simulink model "souk_single_pipeline_4x2"  (R2021a)
settings: Solver=VariableStepAuto  StartTime=0.0  StopTime=10.0  RelTol=1e-3
undefined symbols (not defined in the file): datetime, posixtime
libraries: xbsIndex_r4 x9016, casper_library_misc x75, casper_library_delays x33, casper_library_reorder x22, xps_library x10
(part 16 of 104)

== system souk_single_pipeline_4x2/common/adc_ss/tt_lsb ==
  out_reg : Inport
  assert_reg : xbsIndex_r4/Assert  assert_type=on  type_source=Explicitly  gui_display_data_type=Fixed-point  arith_type=Unsigned  n_bits=32  bin_pt=0  preci_type=Single  exp_width=8  frac_width=24  assert_rate=off  rate_source=Explicitly  period=1  output_port=on  block_type=assert
  cast_gw : xbsIndex_r4/Convert  gui_display_data_type=Fixed-point  arith_type=Unsigned  n_bits=32  bin_pt=0  float_type=Single  exp_bits=8  fraction_bits=24  quantization=Truncate  overflow=Wrap  en=off  latency=1  pipeline=off  dbl_ovrd=off  block_type=convert
  io_delay : xbsIndex_r4/Delay  rst=off  infoeditControl=Selection of Reset will increase slice count due to use of real FFs and instead of SRLs  en=off  latency=0  reg_retiming=on  dbl_ovrd=off  block_type=delay
  reint1 : xbsIndex_r4/Reinterpret  force_arith_type=on  arith_type=Unsigned  force_bin_pt=on  bin_pt=0  block_type=reinterpret
  sim_out : Terminator
  sim_out_reg_gw : xbsIndex_r4/Gateway Out  inherit_from_input=off  hdl_port=off  rows=1  columns=1  UseAsDAC=off  DACChannel='1'  interface=None  automatic_assignment=on  address_offset=hex2dec('00')  intf_name=''  intf_description=''  timing_constraint=None  locs_specified=off  LOCs={}  io_standard={}  block_type=gatewayout
  sim_out_reg_sim_delay : xbsIndex_r4/Delay  rst=off  infoeditControl=Selection of Reset will increase slice count due to use of real FFs and instead of SRLs  en=off  latency=1  reg_retiming=on  dbl_ovrd=off  block_type=delay
  souk_single_pipeline_4x2_common_adc_ss_tt_lsb_user_data_in : xbsIndex_r4/Gateway Out  inherit_from_input=off  hdl_port=on  rows=1  columns=1  UseAsDAC=off  DACChannel='1'  interface=None  automatic_assignment=on  address_offset=hex2dec('00')  intf_name=''  intf_description=''  timing_constraint=None  locs_specified=off  LOCs={}  io_standard={}  block_type=gatewayout
  sim_out_reg : Outport  VectorParamsAs1DForOutWhenUnconnected=off
  wires:
  sim_out_reg_sim_delay/1 -> sim_out_reg_gw/1
  sim_out_reg_gw/1 -> sim_out_reg/1
  io_delay/1 -> cast_gw/1
  cast_gw/1 -> souk_single_pipeline_4x2_common_adc_ss_tt_lsb_user_data_in/1
  souk_single_pipeline_4x2_common_adc_ss_tt_lsb_user_data_in/1 -> sim_out/1
  out_reg/1 -> sim_out_reg_sim_delay/1, assert_reg/1
  assert_reg/1 -> reint1/1
  reint1/1 -> io_delay/1

== system souk_single_pipeline_4x2/common/adc_ss/tt_msb ==
  out_reg : Inport
  assert_reg : xbsIndex_r4/Assert  assert_type=on  type_source=Explicitly  gui_display_data_type=Fixed-point  arith_type=Unsigned  n_bits=32  bin_pt=0  preci_type=Single  exp_width=8  frac_width=24  assert_rate=off  rate_source=Explicitly  period=1  output_port=on  block_type=assert
  cast_gw : xbsIndex_r4/Convert  gui_display_data_type=Fixed-point  arith_type=Unsigned  n_bits=32  bin_pt=0  float_type=Single  exp_bits=8  fraction_bits=24  quantization=Truncate  overflow=Wrap  en=off  latency=1  pipeline=off  dbl_ovrd=off  block_type=convert
  io_delay : xbsIndex_r4/Delay  rst=off  infoeditControl=Selection of Reset will increase slice count due to use of real FFs and instead of SRLs  en=off  latency=0  reg_retiming=on  dbl_ovrd=off  block_type=delay
  reint1 : xbsIndex_r4/Reinterpret  force_arith_type=on  arith_type=Unsigned  force_bin_pt=on  bin_pt=0  block_type=reinterpret
  sim_out : Terminator
  sim_out_reg_gw : xbsIndex_r4/Gateway Out  inherit_from_input=off  hdl_port=off  rows=1  columns=1  UseAsDAC=off  DACChannel='1'  interface=None  automatic_assignment=on  address_offset=hex2dec('00')  intf_name=''  intf_description=''  timing_constraint=None  locs_specified=off  LOCs={}  io_standard={}  block_type=gatewayout
  sim_out_reg_sim_delay : xbsIndex_r4/Delay  rst=off  infoeditControl=Selection of Reset will increase slice count due to use of real FFs and instead of SRLs  en=off  latency=1  reg_retiming=on  dbl_ovrd=off  block_type=delay
  souk_single_pipeline_4x2_common_adc_ss_tt_msb_user_data_in : xbsIndex_r4/Gateway Out  inherit_from_input=off  hdl_port=on  rows=1  columns=1  UseAsDAC=off  DACChannel='1'  interface=None  automatic_assignment=on  address_offset=hex2dec('00')  intf_name=''  intf_description=''  timing_constraint=None  locs_specified=off  LOCs={}  io_standard={}  block_type=gatewayout
  sim_out_reg : Outport  VectorParamsAs1DForOutWhenUnconnected=off
  wires:
  sim_out_reg_sim_delay/1 -> sim_out_reg_gw/1
  sim_out_reg_gw/1 -> sim_out_reg/1
  io_delay/1 -> cast_gw/1
  cast_gw/1 -> souk_single_pipeline_4x2_common_adc_ss_tt_msb_user_data_in/1
  souk_single_pipeline_4x2_common_adc_ss_tt_msb_user_data_in/1 -> sim_out/1
  out_reg/1 -> sim_out_reg_sim_delay/1, assert_reg/1
  assert_reg/1 -> reint1/1
  reint1/1 -> io_delay/1

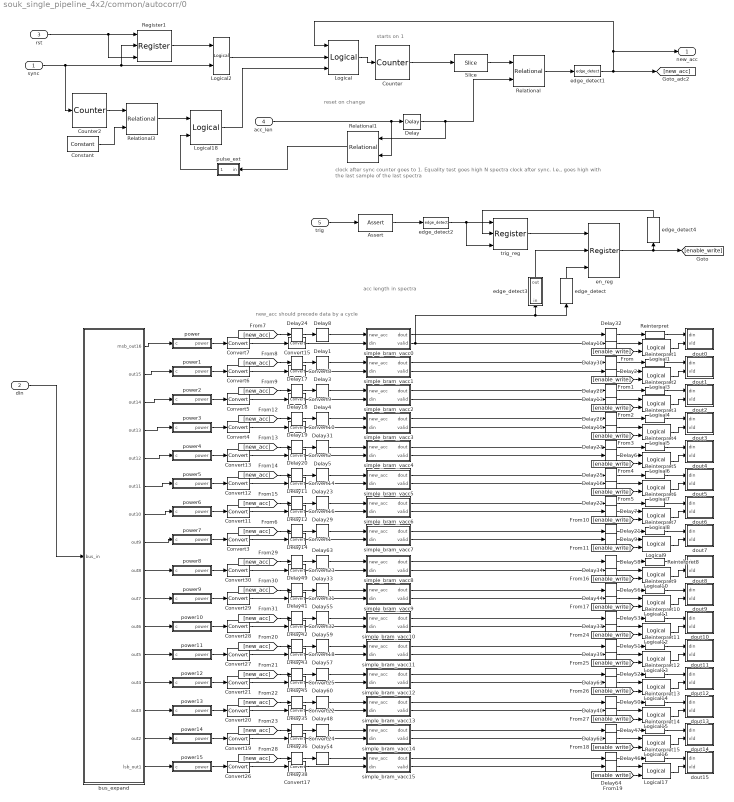
== system souk_single_pipeline_4x2/common/autocorr/0 ==
  note: reset on change
  note: starts on 1
  note: clock after sync counter goes to 1.
      |
      | Equality test goes high N spectra clock after sync. I.e., goes high with the last sample of the last spectra
  note: acc length in spectra
  note: new_acc should precede data by a cycle
  sync : Inport
  din : Inport  Port=2
  rst : Inport  Port=3
  acc_len : Inport  Port=4
  trig : Inport  Port=5
  Assert : xbsIndex_r4/Assert  assert_type=off  type_source=Explicitly  gui_display_data_type=Fixed-point  arith_type="Signed  (2's comp)"  n_bits=16  bin_pt=14  preci_type=Single  exp_width=8  frac_width=24  assert_rate=on  rate_source=Explicitly  period=1  output_port=on  block_type=assert
  Constant : xbsIndex_r4/Constant  const=2^(nchan_bits + npol_bits) - 1  gui_display_data_type=Fixed-point  arith_type=Unsigned  n_bits=nchan_bits + npol_bits  bin_pt=0  preci_type=Single  exp_width=8  frac_width=24  explicit_period=on  period=1  equ=P=C  opselect=C  inp2=PCIN>>17  opr=+  inp1=P  carry=CIN  dbl_ovrd=off  block_type=constant
  Convert{1..2,8..10,14..18,22..25,31..32} (16 alike) : xbsIndex_r4/Convert  gui_display_data_type=Floating-point  arith_type=Floating-point  n_bits=31  bin_pt=28  float_type=Single  exp_bits=8  fraction_bits=24  quantization="Round  (unbiased: Even Values)"  overflow=Wrap  en=off  latency=3  pipeline=on  dbl_ovrd=off  block_type=convert
  Convert{3..7,11..13,19..21,26..30} (16 alike) : xbsIndex_r4/Convert  gui_display_data_type=Fixed-point  arith_type="Signed  (2's comp)"  n_bits=37  bin_pt=34  float_type=Single  exp_bits=8  fraction_bits=24  quantization=Truncate  overflow=Wrap  en=off  latency=0  pipeline=off  dbl_ovrd=off  block_type=convert
  Counter : xbsIndex_r4/Counter  cnt_type=Free Running  cnt_to=Inf  operation=Up  start_count=1  cnt_by_val=1  arith_type=Unsigned  n_bits=30  bin_pt=0  load_pin=off  rst=on  en=off  explicit_period=on  period=1  use_behavioral_HDL=off  implementation=Fabric  dbl_ovrd=off  block_type=counter
  Counter2 : xbsIndex_r4/Counter  cnt_type=Free Running  cnt_to=Inf  operation=Up  start_count=0  cnt_by_val=1  arith_type=Unsigned  n_bits=nchan_bits + npol_bits  bin_pt=0  load_pin=off  rst=on  en=off  explicit_period=on  period=1  use_behavioral_HDL=off  implementation=Fabric  dbl_ovrd=off  block_type=counter
  Delay{,2,6..7,9..10,13,15..16,34,37,39..40,44,61..62,64} (17 alike) : xbsIndex_r4/Delay  rst=off  infoeditControl=Selection of Reset will increase slice count due to use of real FFs and instead of SRLs  en=off  latency=1  reg_retiming=off  dbl_ovrd=off  block_type=delay
  Delay{1,3..5,8,23,29,31,33,48,54..55,57,59..60,63} (16 alike) : xbsIndex_r4/Delay  rst=off  infoeditControl=Selection of Reset will increase slice count due to use of real FFs and instead of SRLs  en=off  latency=4  reg_retiming=on  dbl_ovrd=off  block_type=delay
  Delay{11..12,14,17..20,24,35..36,38,41..43,45,49} (16 alike) : xbsIndex_r4/Delay  rst=off  infoeditControl=Selection of Reset will increase slice count due to use of real FFs and instead of SRLs  en=off  latency=3  reg_retiming=on  dbl_ovrd=off  block_type=delay
  Delay{21..22,25..28,30,32,46..47,50..53,56,58} (16 alike) : xbsIndex_r4/Delay  rst=off  infoeditControl=Selection of Reset will increase slice count due to use of real FFs and instead of SRLs  en=off  latency=1  reg_retiming=on  dbl_ovrd=off  block_type=delay
  Logical : xbsIndex_r4/Logical  logical_function=OR  inputs=3  en=off  latency=0  precision=Full  arith_type=Unsigned  n_bits=16  bin_pt=0  align_bp=on  dbl_ovrd=off  block_type=logical
  Logical{1..18} (18 alike) : xbsIndex_r4/Logical  logical_function=AND  inputs=2  en=off  latency=0  precision=Full  arith_type=Unsigned  n_bits=16  bin_pt=0  align_bp=on  dbl_ovrd=off  block_type=logical
  Register1 : xbsIndex_r4/Register  init=0  rst=on  en=on  dbl_ovrd=off  block_type=register
  Reinterpret{,1..15} (16 alike) : xbsIndex_r4/Reinterpret  force_arith_type=on  arith_type=Unsigned  force_bin_pt=on  bin_pt=0  block_type=reinterpret
  Relational : xbsIndex_r4/Relational  mode=a=b  op_type=Bool  en=off  latency=0  dbl_ovrd=off  block_type=relational
  Relational1 : xbsIndex_r4/Relational  mode=a!=b  op_type=Bool  en=off  latency=1  dbl_ovrd=off  block_type=relational
  Relational3 : xbsIndex_r4/Relational  mode=a=b  op_type=Bool  en=off  latency=1  dbl_ovrd=off  block_type=relational
  Slice : xbsIndex_r4/Slice  nbits=30-nchan_bits-npol_bits  boolean_output=off  mode=Lower Bit Location + Width  bit1=0  base1=MSB of Input  bit0=nchan_bits + npol_bits  base0=LSB of Input  dbl_ovrd=off  block_type=slice
  bus_expand : Subsystem  AncestorBlock=casper_library_flow_control/bus_expand  mask(bus_expand){mode=divisions of equal size, outputNum=16, outputWidth=36, outputBinaryPt=0, outputArithmeticType=0, show_format=off, outputToWorkspace=off, variablePrefix=out, outputToModelAsWell=on}
      mask prompts: outputNum "Number of outputs:"; outputWidth "Output width:"; outputBinaryPt "Output binary point position:"; outputArithmeticType "Output arithmetic type (ufix=0, fix=1, bool=2):"; show_format "Print format string?"; outputToWorkspace "Output to workspace?"; variablePrefix "Variable name prefix:"; outputToModelAsWell "Output to model as well?"
      mask help:
      | Expands a 'bus' made using a bus_create or Xilinx
      | concat block.
      | The input will be divided into the specified number
      | of outputs with the specified arithmetic types.
      | Divisions are made from most significant bit.
      mask init: same as souk_single_pipeline_4x2/bus_expand
      settings: AttributesFormatString=16 outputs
      mask TypeOptions mode: divisions of equal size | divisions of arbitrary size
      mask Callback mode: %bus_expand_callback();
      mask Callback outputWidth: %bus_expand_callback();
      mask Callback outputToWorkspace: %bus_expand_callback();
  dout0 : Subsystem
  dout1 : Subsystem
  dout10 : Subsystem
  dout11 : Subsystem
  dout12 : Subsystem
  dout13 : Subsystem
  dout14 : Subsystem
  dout15 : Subsystem
  dout2 : Subsystem
  dout3 : Subsystem
  dout4 : Subsystem
  dout5 : Subsystem
  dout6 : Subsystem
  dout7 : Subsystem
  dout8 : Subsystem
  dout9 : Subsystem
  edge_detect{,1..2,4} (4 alike) : casper_library_misc/edge_detect  edge=Rising  polarity=Active High  x_in=[0 0.08 0.08 0.16 0.16 0.24 0.24 0.32 0.32 0.4]  y_in="[-1 -1  1  1  1  1  1  1  1  1]"  x_out=[0.6 0.68 0.68 0.76 0.76 0.84 0.84 0.92 0.92 1]  y_out="[-1 -1  1  1 -1 -1 -1 -1 -1 -1]"
  edge_detect3 : Subsystem  AncestorBlock=casper_library_misc/edge_detect  mask(edge_detect){edge=Falling, polarity=Active High, x_in=[0 0.08 0.08 0.16 0.16 0.24 0.24 0.32 0.32 0.4], y_in=[-1 -1  1  1  1  1  1  1  1  1], x_out=[0.6 0.68 0.68 0.76 0.76 0.84 0.84 0.92 0.92 1], y_out=[-1 -1  1  1 -1 -1 -1 -1 -1 -1]}
      mask prompts: edge "Edge Type"; polarity "Output Polarity"; x_in "Input X Positions"; y_in "Input Y Positions"; x_out "Output X Positions"; y_out "Output Y Positions"
      mask help: Output is active for one-cycle after each edge of the specified type (i.e. rising, falling or both).
      mask init: same as souk_single_pipeline_4x2/pulse_ext/posedge
      settings: AttributesFormatString=|
      | falling edges
      | active high
      mask Help: Output is active for one-cycle after each edge of the specified type (i.e. rising, falling, or both).  Latency is zero.
      mask TypeOptions edge: Rising | Falling | Both
      mask TypeOptions polarity: Active High | Active Low
      mask Display:
      | plot(x_in_num,0.5+y_in_num*0.2);
      | plot(x_out_num,0.5+y_out_num*0.2);
  en_reg : xbsIndex_r4/Register  init=0  rst=on  en=on  dbl_ovrd=off  block_type=register
  power : Subsystem  mask(power){BitWidth=18, add_latency=1, mult_latency=3}
      mask prompts: BitWidth "Bit Width"; add_latency "Add Latency"; mult_latency "Mult Latency"
      mask help: Squares real and imaginary components of complex input and adds them.
      mask Help: eval('xlWeb(''http://casper.berkeley.edu/wiki/Power'')')
      mask Display:
      | port_label('input', 1, 'c');
      | port_label('output', 1, 'power');
      | disp(['Z^-', num2str(mult_latency+add_latency)]);
  power1 : Subsystem  mask(power){BitWidth=18, add_latency=1, mult_latency=3}
      mask prompts: BitWidth "Bit Width"; add_latency "Add Latency"; mult_latency "Mult Latency"
      mask help: Squares real and imaginary components of complex input and adds them.
      mask Help: eval('xlWeb(''http://casper.berkeley.edu/wiki/Power'')')
      mask Display:
      | port_label('input', 1, 'c');
      | port_label('output', 1, 'power');
      | disp(['Z^-', num2str(mult_latency+add_latency)]);
  power10 : Subsystem  mask(power){BitWidth=18, add_latency=1, mult_latency=3}
      mask prompts: BitWidth "Bit Width"; add_latency "Add Latency"; mult_latency "Mult Latency"
      mask help: Squares real and imaginary components of complex input and adds them.
      mask Help: eval('xlWeb(''http://casper.berkeley.edu/wiki/Power'')')
      mask Display:
      | port_label('input', 1, 'c');
      | port_label('output', 1, 'power');
      | disp(['Z^-', num2str(mult_latency+add_latency)]);
  power11 : Subsystem  mask(power){BitWidth=18, add_latency=1, mult_latency=3}
      mask prompts: BitWidth "Bit Width"; add_latency "Add Latency"; mult_latency "Mult Latency"
      mask help: Squares real and imaginary components of complex input and adds them.
      mask Help: eval('xlWeb(''http://casper.berkeley.edu/wiki/Power'')')
      mask Display:
      | port_label('input', 1, 'c');
      | port_label('output', 1, 'power');
      | disp(['Z^-', num2str(mult_latency+add_latency)]);
  power12 : Subsystem  mask(power){BitWidth=18, add_latency=1, mult_latency=3}
      mask prompts: BitWidth "Bit Width"; add_latency "Add Latency"; mult_latency "Mult Latency"
      mask help: Squares real and imaginary components of complex input and adds them.
      mask Help: eval('xlWeb(''http://casper.berkeley.edu/wiki/Power'')')
      mask Display:
      | port_label('input', 1, 'c');
      | port_label('output', 1, 'power');
      | disp(['Z^-', num2str(mult_latency+add_latency)]);
  power13 : Subsystem  mask(power){BitWidth=18, add_latency=1, mult_latency=3}
      mask prompts: BitWidth "Bit Width"; add_latency "Add Latency"; mult_latency "Mult Latency"
      mask help: Squares real and imaginary components of complex input and adds them.
      mask Help: eval('xlWeb(''http://casper.berkeley.edu/wiki/Power'')')
      mask Display:
      | port_label('input', 1, 'c');
      | port_label('output', 1, 'power');
      | disp(['Z^-', num2str(mult_latency+add_latency)]);
  power14 : Subsystem  mask(power){BitWidth=18, add_latency=1, mult_latency=3}
      mask prompts: BitWidth "Bit Width"; add_latency "Add Latency"; mult_latency "Mult Latency"
      mask help: Squares real and imaginary components of complex input and adds them.
      mask Help: eval('xlWeb(''http://casper.berkeley.edu/wiki/Power'')')
      mask Display:
      | port_label('input', 1, 'c');
      | port_label('output', 1, 'power');
      | disp(['Z^-', num2str(mult_latency+add_latency)]);
  power15 : Subsystem  mask(power){BitWidth=18, add_latency=1, mult_latency=3}
      mask prompts: BitWidth "Bit Width"; add_latency "Add Latency"; mult_latency "Mult Latency"
      mask help: Squares real and imaginary components of complex input and adds them.
      mask Help: eval('xlWeb(''http://casper.berkeley.edu/wiki/Power'')')
      mask Display:
      | port_label('input', 1, 'c');
      | port_label('output', 1, 'power');
      | disp(['Z^-', num2str(mult_latency+add_latency)]);
  power2 : Subsystem  mask(power){BitWidth=18, add_latency=1, mult_latency=3}
      mask prompts: BitWidth "Bit Width"; add_latency "Add Latency"; mult_latency "Mult Latency"
      mask help: Squares real and imaginary components of complex input and adds them.
      mask Help: eval('xlWeb(''http://casper.berkeley.edu/wiki/Power'')')
      mask Display:
      | port_label('input', 1, 'c');
      | port_label('output', 1, 'power');
      | disp(['Z^-', num2str(mult_latency+add_latency)]);
  power3 : Subsystem  mask(power){BitWidth=18, add_latency=1, mult_latency=3}
      mask prompts: BitWidth "Bit Width"; add_latency "Add Latency"; mult_latency "Mult Latency"
      mask help: Squares real and imaginary components of complex input and adds them.
      mask Help: eval('xlWeb(''http://casper.berkeley.edu/wiki/Power'')')
      mask Display:
      | port_label('input', 1, 'c');
      | port_label('output', 1, 'power');
      | disp(['Z^-', num2str(mult_latency+add_latency)]);
  power4 : Subsystem  mask(power){BitWidth=18, add_latency=1, mult_latency=3}
      mask prompts: BitWidth "Bit Width"; add_latency "Add Latency"; mult_latency "Mult Latency"
      mask help: Squares real and imaginary components of complex input and adds them.
      mask Help: eval('xlWeb(''http://casper.berkeley.edu/wiki/Power'')')
      mask Display:
      | port_label('input', 1, 'c');
      | port_label('output', 1, 'power');
      | disp(['Z^-', num2str(mult_latency+add_latency)]);
  power5 : Subsystem  mask(power){BitWidth=18, add_latency=1, mult_latency=3}
      mask prompts: BitWidth "Bit Width"; add_latency "Add Latency"; mult_latency "Mult Latency"
      mask help: Squares real and imaginary components of complex input and adds them.
      mask Help: eval('xlWeb(''http://casper.berkeley.edu/wiki/Power'')')
      mask Display:
      | port_label('input', 1, 'c');
      | port_label('output', 1, 'power');
      | disp(['Z^-', num2str(mult_latency+add_latency)]);
  power6 : Subsystem  mask(power){BitWidth=18, add_latency=1, mult_latency=3}
      mask prompts: BitWidth "Bit Width"; add_latency "Add Latency"; mult_latency "Mult Latency"
      mask help: Squares real and imaginary components of complex input and adds them.
      mask Help: eval('xlWeb(''http://casper.berkeley.edu/wiki/Power'')')
      mask Display:
      | port_label('input', 1, 'c');
      | port_label('output', 1, 'power');
      | disp(['Z^-', num2str(mult_latency+add_latency)]);
  power7 : Subsystem  mask(power){BitWidth=18, add_latency=1, mult_latency=3}
      mask prompts: BitWidth "Bit Width"; add_latency "Add Latency"; mult_latency "Mult Latency"
      mask help: Squares real and imaginary components of complex input and adds them.
      mask Help: eval('xlWeb(''http://casper.berkeley.edu/wiki/Power'')')
      mask Display:
      | port_label('input', 1, 'c');
      | port_label('output', 1, 'power');
      | disp(['Z^-', num2str(mult_latency+add_latency)]);
  power8 : Subsystem  mask(power){BitWidth=18, add_latency=1, mult_latency=3}
      mask prompts: BitWidth "Bit Width"; add_latency "Add Latency"; mult_latency "Mult Latency"
      mask help: Squares real and imaginary components of complex input and adds them.
      mask Help: eval('xlWeb(''http://casper.berkeley.edu/wiki/Power'')')
      mask Display:
      | port_label('input', 1, 'c');
      | port_label('output', 1, 'power');
      | disp(['Z^-', num2str(mult_latency+add_latency)]);
  power9 : Subsystem  mask(power){BitWidth=18, add_latency=1, mult_latency=3}
      mask prompts: BitWidth "Bit Width"; add_latency "Add Latency"; mult_latency "Mult Latency"
      mask help: Squares real and imaginary components of complex input and adds them.
      mask Help: eval('xlWeb(''http://casper.berkeley.edu/wiki/Power'')')
      mask Display:
      | port_label('input', 1, 'c');
      | port_label('output', 1, 'power');
      | disp(['Z^-', num2str(mult_latency+add_latency)]);
  pulse_ext : Subsystem  AncestorBlock=casper_library_misc/pulse_ext  mask(pulse_ext){pulse_len=2^(nchan_bits + npol_bits)}
      mask prompts: pulse_len "Length of Pulse"
      mask help:
      | Extends a boolean signal to be high for the specified number of clocks after
      | the last high input.
      mask init:
      | bits = ceil(log2(pulse_len+1));
      mask Help: eval('xlWeb(''http://casper.berkeley.edu/wiki/Pulse_ext'')')
  simple_bram_vacc0 : Subsystem  AncestorBlock=casper_library_accumulators/simple_bram_vacc  mask(simple_bram_vacc){vec_len=2^(nchan_bits + npol_bits), arith_type=Signed, n_bits=30 + 17, bin_pt=28}
      mask prompts: vec_len "Vector length:"; arith_type "Output type:"; n_bits "Bit width (output):"; bin_pt "Binary point (output):"
      mask help: This simple vector accumulator is based on a shift register. It outputs its previous accumulated vector after a new_acc pulse is received.
      mask init:
      | simple_bram_vacc_init(gcb, ...
      |     'vec_len', vec_len, ...
      |     'arith_type', arith_type, ...
      |     'n_bits', n_bits, ...
      |     'bin_pt', bin_pt);
      mask TypeOptions arith_type: Signed | Unsigned
  simple_bram_vacc1 : Subsystem  AncestorBlock=casper_library_accumulators/simple_bram_vacc  mask(simple_bram_vacc){vec_len=2^(nchan_bits + npol_bits), arith_type=Signed, n_bits=30 + 17, bin_pt=28}
      mask prompts: vec_len "Vector length:"; arith_type "Output type:"; n_bits "Bit width (output):"; bin_pt "Binary point (output):"
      mask help: This simple vector accumulator is based on a shift register. It outputs its previous accumulated vector after a new_acc pulse is received.
      mask init:
      | simple_bram_vacc_init(gcb, ...
      |     'vec_len', vec_len, ...
      |     'arith_type', arith_type, ...
      |     'n_bits', n_bits, ...
      |     'bin_pt', bin_pt);
      mask TypeOptions arith_type: Signed | Unsigned
  simple_bram_vacc10 : Subsystem  AncestorBlock=casper_library_accumulators/simple_bram_vacc  mask(simple_bram_vacc){vec_len=2^(nchan_bits + npol_bits), arith_type=Signed, n_bits=30 + 17, bin_pt=28}
      mask prompts: vec_len "Vector length:"; arith_type "Output type:"; n_bits "Bit width (output):"; bin_pt "Binary point (output):"
      mask help: This simple vector accumulator is based on a shift register. It outputs its previous accumulated vector after a new_acc pulse is received.
      mask init:
      | simple_bram_vacc_init(gcb, ...
      |     'vec_len', vec_len, ...
      |     'arith_type', arith_type, ...
      |     'n_bits', n_bits, ...
      |     'bin_pt', bin_pt);
      mask TypeOptions arith_type: Signed | Unsigned
  simple_bram_vacc11 : Subsystem  AncestorBlock=casper_library_accumulators/simple_bram_vacc  mask(simple_bram_vacc){vec_len=2^(nchan_bits + npol_bits), arith_type=Signed, n_bits=30 + 17, bin_pt=28}
      mask prompts: vec_len "Vector length:"; arith_type "Output type:"; n_bits "Bit width (output):"; bin_pt "Binary point (output):"
      mask help: This simple vector accumulator is based on a shift register. It outputs its previous accumulated vector after a new_acc pulse is received.
      mask init:
      | simple_bram_vacc_init(gcb, ...
      |     'vec_len', vec_len, ...
      |     'arith_type', arith_type, ...
      |     'n_bits', n_bits, ...
      |     'bin_pt', bin_pt);
      mask TypeOptions arith_type: Signed | Unsigned
  simple_bram_vacc12 : Subsystem  AncestorBlock=casper_library_accumulators/simple_bram_vacc  mask(simple_bram_vacc){vec_len=2^(nchan_bits + npol_bits), arith_type=Signed, n_bits=30 + 17, bin_pt=28}
      mask prompts: vec_len "Vector length:"; arith_type "Output type:"; n_bits "Bit width (output):"; bin_pt "Binary point (output):"
      mask help: This simple vector accumulator is based on a shift register. It outputs its previous accumulated vector after a new_acc pulse is received.
      mask init:
      | simple_bram_vacc_init(gcb, ...
      |     'vec_len', vec_len, ...
      |     'arith_type', arith_type, ...
      |     'n_bits', n_bits, ...
      |     'bin_pt', bin_pt);
      mask TypeOptions arith_type: Signed | Unsigned
  simple_bram_vacc13 : Subsystem  AncestorBlock=casper_library_accumulators/simple_bram_vacc  mask(simple_bram_vacc){vec_len=2^(nchan_bits + npol_bits), arith_type=Signed, n_bits=30 + 17, bin_pt=28}
      mask prompts: vec_len "Vector length:"; arith_type "Output type:"; n_bits "Bit width (output):"; bin_pt "Binary point (output):"
      mask help: This simple vector accumulator is based on a shift register. It outputs its previous accumulated vector after a new_acc pulse is received.
      mask init:
      | simple_bram_vacc_init(gcb, ...
      |     'vec_len', vec_len, ...
      |     'arith_type', arith_type, ...
      |     'n_bits', n_bits, ...
      |     'bin_pt', bin_pt);
      mask TypeOptions arith_type: Signed | Unsigned
  simple_bram_vacc14 : Subsystem  AncestorBlock=casper_library_accumulators/simple_bram_vacc  mask(simple_bram_vacc){vec_len=2^(nchan_bits + npol_bits), arith_type=Signed, n_bits=30 + 17, bin_pt=28}
      mask prompts: vec_len "Vector length:"; arith_type "Output type:"; n_bits "Bit width (output):"; bin_pt "Binary point (output):"
      mask help: This simple vector accumulator is based on a shift register. It outputs its previous accumulated vector after a new_acc pulse is received.
      mask init:
      | simple_bram_vacc_init(gcb, ...
      |     'vec_len', vec_len, ...
      |     'arith_type', arith_type, ...
      |     'n_bits', n_bits, ...
      |     'bin_pt', bin_pt);
      mask TypeOptions arith_type: Signed | Unsigned
  simple_bram_vacc15 : Subsystem  AncestorBlock=casper_library_accumulators/simple_bram_vacc  mask(simple_bram_vacc){vec_len=2^(nchan_bits + npol_bits), arith_type=Signed, n_bits=30 + 17, bin_pt=28}
      mask prompts: vec_len "Vector length:"; arith_type "Output type:"; n_bits "Bit width (output):"; bin_pt "Binary point (output):"
      mask help: This simple vector accumulator is based on a shift register. It outputs its previous accumulated vector after a new_acc pulse is received.
      mask init:
      | simple_bram_vacc_init(gcb, ...
      |     'vec_len', vec_len, ...
      |     'arith_type', arith_type, ...
      |     'n_bits', n_bits, ...
      |     'bin_pt', bin_pt);
      mask TypeOptions arith_type: Signed | Unsigned
  simple_bram_vacc2 : Subsystem  AncestorBlock=casper_library_accumulators/simple_bram_vacc  mask(simple_bram_vacc){vec_len=2^(nchan_bits + npol_bits), arith_type=Signed, n_bits=30 + 17, bin_pt=28}
      mask prompts: vec_len "Vector length:"; arith_type "Output type:"; n_bits "Bit width (output):"; bin_pt "Binary point (output):"
      mask help: This simple vector accumulator is based on a shift register. It outputs its previous accumulated vector after a new_acc pulse is received.
      mask init:
      | simple_bram_vacc_init(gcb, ...
      |     'vec_len', vec_len, ...
      |     'arith_type', arith_type, ...
      |     'n_bits', n_bits, ...
      |     'bin_pt', bin_pt);
      mask TypeOptions arith_type: Signed | Unsigned
  simple_bram_vacc3 : Subsystem  AncestorBlock=casper_library_accumulators/simple_bram_vacc  mask(simple_bram_vacc){vec_len=2^(nchan_bits + npol_bits), arith_type=Signed, n_bits=30 + 17, bin_pt=28}
      mask prompts: vec_len "Vector length:"; arith_type "Output type:"; n_bits "Bit width (output):"; bin_pt "Binary point (output):"
      mask help: This simple vector accumulator is based on a shift register. It outputs its previous accumulated vector after a new_acc pulse is received.
      mask init:
      | simple_bram_vacc_init(gcb, ...
      |     'vec_len', vec_len, ...
      |     'arith_type', arith_type, ...
      |     'n_bits', n_bits, ...
      |     'bin_pt', bin_pt);
      mask TypeOptions arith_type: Signed | Unsigned
  simple_bram_vacc4 : Subsystem  AncestorBlock=casper_library_accumulators/simple_bram_vacc  mask(simple_bram_vacc){vec_len=2^(nchan_bits + npol_bits), arith_type=Signed, n_bits=30 + 17, bin_pt=28}
      mask prompts: vec_len "Vector length:"; arith_type "Output type:"; n_bits "Bit width (output):"; bin_pt "Binary point (output):"
      mask help: This simple vector accumulator is based on a shift register. It outputs its previous accumulated vector after a new_acc pulse is received.
      mask init:
      | simple_bram_vacc_init(gcb, ...
      |     'vec_len', vec_len, ...
      |     'arith_type', arith_type, ...
      |     'n_bits', n_bits, ...
      |     'bin_pt', bin_pt);
      mask TypeOptions arith_type: Signed | Unsigned
  simple_bram_vacc5 : Subsystem  AncestorBlock=casper_library_accumulators/simple_bram_vacc  mask(simple_bram_vacc){vec_len=2^(nchan_bits + npol_bits), arith_type=Signed, n_bits=30 + 17, bin_pt=28}
      mask prompts: vec_len "Vector length:"; arith_type "Output type:"; n_bits "Bit width (output):"; bin_pt "Binary point (output):"
      mask help: This simple vector accumulator is based on a shift register. It outputs its previous accumulated vector after a new_acc pulse is received.
      mask init:
      | simple_bram_vacc_init(gcb, ...
      |     'vec_len', vec_len, ...
      |     'arith_type', arith_type, ...
      |     'n_bits', n_bits, ...
      |     'bin_pt', bin_pt);
      mask TypeOptions arith_type: Signed | Unsigned
  simple_bram_vacc6 : Subsystem  AncestorBlock=casper_library_accumulators/simple_bram_vacc  mask(simple_bram_vacc){vec_len=2^(nchan_bits + npol_bits), arith_type=Signed, n_bits=30 + 17, bin_pt=28}
      mask prompts: vec_len "Vector length:"; arith_type "Output type:"; n_bits "Bit width (output):"; bin_pt "Binary point (output):"
      mask help: This simple vector accumulator is based on a shift register. It outputs its previous accumulated vector after a new_acc pulse is received.
      mask init:
      | simple_bram_vacc_init(gcb, ...
      |     'vec_len', vec_len, ...
      |     'arith_type', arith_type, ...
      |     'n_bits', n_bits, ...
      |     'bin_pt', bin_pt);
      mask TypeOptions arith_type: Signed | Unsigned
  simple_bram_vacc7 : Subsystem  AncestorBlock=casper_library_accumulators/simple_bram_vacc  mask(simple_bram_vacc){vec_len=2^(nchan_bits + npol_bits), arith_type=Signed, n_bits=30 + 17, bin_pt=28}
      mask prompts: vec_len "Vector length:"; arith_type "Output type:"; n_bits "Bit width (output):"; bin_pt "Binary point (output):"
      mask help: This simple vector accumulator is based on a shift register. It outputs its previous accumulated vector after a new_acc pulse is received.
      mask init:
      | simple_bram_vacc_init(gcb, ...
      |     'vec_len', vec_len, ...
      |     'arith_type', arith_type, ...
      |     'n_bits', n_bits, ...
      |     'bin_pt', bin_pt);
      mask TypeOptions arith_type: Signed | Unsigned
  simple_bram_vacc8 : Subsystem  AncestorBlock=casper_library_accumulators/simple_bram_vacc  mask(simple_bram_vacc){vec_len=2^(nchan_bits + npol_bits), arith_type=Signed, n_bits=30 + 17, bin_pt=28}
      mask prompts: vec_len "Vector length:"; arith_type "Output type:"; n_bits "Bit width (output):"; bin_pt "Binary point (output):"
      mask help: This simple vector accumulator is based on a shift register. It outputs its previous accumulated vector after a new_acc pulse is received.
      mask init:
      | simple_bram_vacc_init(gcb, ...
      |     'vec_len', vec_len, ...
      |     'arith_type', arith_type, ...
      |     'n_bits', n_bits, ...
      |     'bin_pt', bin_pt);
      mask TypeOptions arith_type: Signed | Unsigned
  simple_bram_vacc9 : Subsystem  AncestorBlock=casper_library_accumulators/simple_bram_vacc  mask(simple_bram_vacc){vec_len=2^(nchan_bits + npol_bits), arith_type=Signed, n_bits=30 + 17, bin_pt=28}
      mask prompts: vec_len "Vector length:"; arith_type "Output type:"; n_bits "Bit width (output):"; bin_pt "Binary point (output):"
      mask help: This simple vector accumulator is based on a shift register. It outputs its previous accumulated vector after a new_acc pulse is received.
      mask init:
      | simple_bram_vacc_init(gcb, ...
      |     'vec_len', vec_len, ...
      |     'arith_type', arith_type, ...
      |     'n_bits', n_bits, ...
      |     'bin_pt', bin_pt);
      mask TypeOptions arith_type: Signed | Unsigned
  trig_reg : xbsIndex_r4/Register  init=0  rst=on  en=on  dbl_ovrd=off  block_type=register
  new_acc : Outport  VectorParamsAs1DForOutWhenUnconnected=off
  wires:
  Delay/1 -> Relational1/1, Relational/2
  Delay8/1 -> simple_bram_vacc0/1(new_acc)
  Delay1/1 -> simple_bram_vacc1/1(new_acc)
  Delay3/1 -> simple_bram_vacc2/1(new_acc)
  Delay4/1 -> simple_bram_vacc3/1(new_acc)
  acc_len/1 -> Relational1/2, Delay/1
  Logical2/1 -> Logical/2
  Relational/1 -> edge_detect1/1
  Slice/1 -> Relational/1
  din/1 -> bus_expand/1(bus_in)
  power3/1(power) -> Convert4/1
  power2/1(power) -> Convert5/1
  power1/1(power) -> Convert6/1
  power/1(power) -> Convert7/1
  [new_acc] -> Delay19/1
  [new_acc] -> Delay18/1
  [new_acc] -> Delay17/1
  [new_acc] -> Delay24/1
  Counter/1 -> Slice/1
  Logical/1 -> Counter/1
  edge_detect1/1 -> [new_acc], new_acc/1, Logical/1
  rst/1 -> Register1/1, Register1/3
  Register1/1 -> Logical2/1
  trig_reg/1 -> en_reg/1
  edge_detect2/1 -> trig_reg/3, trig_reg/1
  edge_detect/1 -> en_reg/3
  edge_detect3/1(out) -> en_reg/2
  edge_detect4/1 -> trig_reg/2
  Logical1/1 -> dout0/2(vld)
  en_reg/1 -> [enable_write], edge_detect4/1
  [enable_write] -> Logical1/2
  [enable_write] -> Logical3/2
  Logical3/1 -> dout1/2(vld)
  Logical4/1 -> dout2/2(vld)
  [enable_write] -> Logical4/2
  [enable_write] -> Logical5/2
  Logical5/1 -> dout3/2(vld)
  trig/1 -> Assert/1
  Assert/1 -> edge_detect2/1
  simple_bram_vacc0/1(dout) -> Delay32/1
  simple_bram_vacc1/1(dout) -> Delay30/1
  simple_bram_vacc2/1(dout) -> Delay28/1
  simple_bram_vacc2/2(valid) -> Delay13/1
  simple_bram_vacc3/1(dout) -> Delay26/1
  simple_bram_vacc3/2(valid) -> Delay15/1
  simple_bram_vacc1/2(valid) -> Delay2/1
  simple_bram_vacc0/2(valid) -> Delay10/1, edge_detect/1, edge_detect3/1(in)
  Delay19/1 -> Delay4/1
  Convert10/1 -> simple_bram_vacc3/2(din)
  Delay18/1 -> Delay3/1
  Convert9/1 -> simple_bram_vacc2/2(din)
  Convert8/1 -> simple_bram_vacc1/2(din)
  Delay17/1 -> Delay1/1
  Delay24/1 -> Delay8/1
  Convert15/1 -> simple_bram_vacc0/2(din)
  Delay32/1 -> Reinterpret/1
  Delay10/1 -> Logical1/1
  Delay30/1 -> Reinterpret1/1
  Delay2/1 -> Logical3/1
  Delay28/1 -> Reinterpret2/1
  Delay13/1 -> Logical4/1
  Delay15/1 -> Logical5/1
  Delay26/1 -> Reinterpret3/1
  Convert4/1 -> Convert10/1
  Convert5/1 -> Convert9/1
  Convert6/1 -> Convert8/1
  Convert7/1 -> Convert15/1
  Reinterpret/1 -> dout0/1(din)
  Reinterpret1/1 -> dout1/1(din)
  Reinterpret2/1 -> dout2/1(din)
  Reinterpret3/1 -> dout3/1(din)
  Reinterpret7/1 -> dout7/1(din)
  Reinterpret6/1 -> dout6/1(din)
  Reinterpret5/1 -> dout5/1(din)
  Reinterpret4/1 -> dout4/1(din)
  Convert13/1 -> Convert2/1
  Convert12/1 -> Convert14/1
  Convert11/1 -> Convert16/1
  Convert3/1 -> Convert1/1
  Delay21/1 -> Reinterpret7/1
  Delay9/1 -> Logical9/1
  Delay7/1 -> Logical8/1
  Delay22/1 -> Reinterpret6/1
  Delay16/1 -> Logical7/1
  Delay25/1 -> Reinterpret5/1
  Delay6/1 -> Logical6/1
  Delay27/1 -> Reinterpret4/1
  Convert2/1 -> simple_bram_vacc4/2(din)
  Delay20/1 -> Delay31/1
  Delay11/1 -> Delay5/1
  Convert14/1 -> simple_bram_vacc5/2(din)
  Convert16/1 -> simple_bram_vacc6/2(din)
  Delay12/1 -> Delay23/1
  Convert1/1 -> simple_bram_vacc7/2(din)
  Delay14/1 -> Delay29/1
  simple_bram_vacc4/2(valid) -> Delay6/1
  simple_bram_vacc5/2(valid) -> Delay16/1
  simple_bram_vacc7/2(valid) -> Delay9/1
  simple_bram_vacc7/1(dout) -> Delay21/1
  simple_bram_vacc6/2(valid) -> Delay7/1
  simple_bram_vacc6/1(dout) -> Delay22/1
  simple_bram_vacc5/1(dout) -> Delay25/1
  simple_bram_vacc4/1(dout) -> Delay27/1
  Logical9/1 -> dout7/2(vld)
  [enable_write] -> Logical9/2
  [enable_write] -> Logical8/2
  Logical8/1 -> dout6/2(vld)
  Logical7/1 -> dout5/2(vld)
  [enable_write] -> Logical7/2
  [enable_write] -> Logical6/2
  Logical6/1 -> dout4/2(vld)
  [new_acc] -> Delay20/1
  [new_acc] -> Delay11/1
  [new_acc] -> Delay12/1
  [new_acc] -> Delay14/1
  power4/1(power) -> Convert13/1
  power5/1(power) -> Convert12/1
  power6/1(power) -> Convert11/1
  power7/1(power) -> Convert3/1
  Delay29/1 -> simple_bram_vacc7/1(new_acc)
  Delay23/1 -> simple_bram_vacc6/1(new_acc)
  Delay5/1 -> simple_bram_vacc5/1(new_acc)
  Delay31/1 -> simple_bram_vacc4/1(new_acc)
  Delay57/1 -> simple_bram_vacc12/1(new_acc)
  Delay60/1 -> simple_bram_vacc13/1(new_acc)
  Delay48/1 -> simple_bram_vacc14/1(new_acc)
  Delay54/1 -> simple_bram_vacc15/1(new_acc)
  power15/1(power) -> Convert26/1
  power14/1(power) -> Convert19/1
  power13/1(power) -> Convert20/1
  power12/1(power) -> Convert21/1
  [new_acc] -> Delay38/1
  [new_acc] -> Delay36/1
  [new_acc] -> Delay35/1
  [new_acc] -> Delay45/1
  Logical14/1 -> dout12/2(vld)
  [enable_write] -> Logical14/2
  [enable_write] -> Logical15/2
  Logical15/1 -> dout13/2(vld)
  Logical16/1 -> dout14/2(vld)
  [enable_write] -> Logical16/2
  [enable_write] -> Logical17/2
  Logical17/1 -> dout15/2(vld)
  simple_bram_vacc12/1(dout) -> Delay52/1
  simple_bram_vacc13/1(dout) -> Delay50/1
  simple_bram_vacc14/1(dout) -> Delay47/1
  simple_bram_vacc14/2(valid) -> Delay62/1
  simple_bram_vacc15/1(dout) -> Delay46/1
  simple_bram_vacc15/2(valid) -> Delay64/1
  simple_bram_vacc13/2(valid) -> Delay40/1
  simple_bram_vacc12/2(valid) -> Delay61/1
  Delay38/1 -> Delay54/1
  Convert17/1 -> simple_bram_vacc15/2(din)
  Delay36/1 -> Delay48/1
  Convert24/1 -> simple_bram_vacc14/2(din)
  Convert22/1 -> simple_bram_vacc13/2(din)
  Delay35/1 -> Delay60/1
  Delay45/1 -> Delay57/1
  Convert25/1 -> simple_bram_vacc12/2(din)
  Delay52/1 -> Reinterpret12/1
  Delay61/1 -> Logical14/1
  Delay50/1 -> Reinterpret13/1
  Delay40/1 -> Logical15/1
  Delay47/1 -> Reinterpret14/1
  Delay62/1 -> Logical16/1
  Delay64/1 -> Logical17/1
  Delay46/1 -> Reinterpret15/1
  Convert26/1 -> Convert17/1
  Convert19/1 -> Convert24/1
  Convert20/1 -> Convert22/1
  Convert21/1 -> Convert25/1
  Reinterpret12/1 -> dout12/1(din)
  Reinterpret13/1 -> dout13/1(din)
  Reinterpret14/1 -> dout14/1(din)
  Reinterpret15/1 -> dout15/1(din)
  Reinterpret11/1 -> dout11/1(din)
  Reinterpret10/1 -> dout10/1(din)
  Reinterpret9/1 -> dout9/1(din)
  Reinterpret8/1 -> dout8/1(din)
  Convert30/1 -> Convert23/1
  Convert29/1 -> Convert31/1
  Convert28/1 -> Convert32/1
  Convert27/1 -> Convert18/1
  Delay51/1 -> Reinterpret11/1
  Delay39/1 -> Logical13/1
  Delay37/1 -> Logical12/1
  Delay53/1 -> Reinterpret10/1
  Delay44/1 -> Logical11/1
  Delay56/1 -> Reinterpret9/1
  Delay34/1 -> Logical10/1
  Delay58/1 -> Reinterpret8/1
  Convert23/1 -> simple_bram_vacc8/2(din)
  Delay49/1 -> Delay63/1
  Delay41/1 -> Delay33/1
  Convert31/1 -> simple_bram_vacc9/2(din)
  Convert32/1 -> simple_bram_vacc10/2(din)
  Delay42/1 -> Delay55/1
  Convert18/1 -> simple_bram_vacc11/2(din)
  Delay43/1 -> Delay59/1
  simple_bram_vacc8/2(valid) -> Delay34/1
  simple_bram_vacc9/2(valid) -> Delay44/1
  simple_bram_vacc11/2(valid) -> Delay39/1
  simple_bram_vacc11/1(dout) -> Delay51/1
  simple_bram_vacc10/2(valid) -> Delay37/1
  simple_bram_vacc10/1(dout) -> Delay53/1
  simple_bram_vacc9/1(dout) -> Delay56/1
  simple_bram_vacc8/1(dout) -> Delay58/1
  Logical13/1 -> dout11/2(vld)
  [enable_write] -> Logical13/2
  [enable_write] -> Logical12/2
  Logical12/1 -> dout10/2(vld)
  Logical11/1 -> dout9/2(vld)
  [enable_write] -> Logical11/2
  [enable_write] -> Logical10/2
  Logical10/1 -> dout8/2(vld)
  [new_acc] -> Delay49/1
  [new_acc] -> Delay41/1
  [new_acc] -> Delay42/1
  [new_acc] -> Delay43/1
  power8/1(power) -> Convert30/1
  power9/1(power) -> Convert29/1
  power10/1(power) -> Convert28/1
  power11/1(power) -> Convert27/1
  Delay59/1 -> simple_bram_vacc11/1(new_acc)
  Delay55/1 -> simple_bram_vacc10/1(new_acc)
  Delay33/1 -> simple_bram_vacc9/1(new_acc)
  Delay63/1 -> simple_bram_vacc8/1(new_acc)
  bus_expand/9(out8) -> power8/1(c)
  bus_expand/10(out7) -> power9/1(c)
  bus_expand/11(out6) -> power10/1(c)
  bus_expand/12(out5) -> power11/1(c)
  bus_expand/13(out4) -> power12/1(c)
  bus_expand/14(out3) -> power13/1(c)
  bus_expand/15(out2) -> power14/1(c)
  bus_expand/16(lsb_out1) -> power15/1(c)
  bus_expand/1(msb_out16) -> power/1(c)
  bus_expand/2(out15) -> power1/1(c)
  bus_expand/3(out14) -> power2/1(c)
  bus_expand/4(out13) -> power3/1(c)
  bus_expand/5(out12) -> power4/1(c)
  bus_expand/6(out11) -> power5/1(c)
  bus_expand/7(out10) -> power6/1(c)
  bus_expand/8(out9) -> power7/1(c)
  sync/1 -> Counter2/1, Logical2/2, Register1/2
  Counter2/1 -> Relational3/1
  pulse_ext/1(out) -> Logical18/2
  Relational3/1 -> Logical18/1
  Constant/1 -> Relational3/2
  Relational1/1 -> pulse_ext/1(in)
  Logical18/1 -> Logical/3

== system souk_single_pipeline_4x2/common/autocorr/acc_cnt ==
  out_reg : Inport
  assert_reg : xbsIndex_r4/Assert  assert_type=on  type_source=Explicitly  gui_display_data_type=Fixed-point  arith_type=Unsigned  n_bits=32  bin_pt=0  preci_type=Single  exp_width=8  frac_width=24  assert_rate=off  rate_source=Explicitly  period=1  output_port=on  block_type=assert
  cast_gw : xbsIndex_r4/Convert  gui_display_data_type=Fixed-point  arith_type=Unsigned  n_bits=32  bin_pt=0  float_type=Single  exp_bits=8  fraction_bits=24  quantization=Truncate  overflow=Wrap  en=off  latency=1  pipeline=off  dbl_ovrd=off  block_type=convert
  io_delay : xbsIndex_r4/Delay  rst=off  infoeditControl=Selection of Reset will increase slice count due to use of real FFs and instead of SRLs  en=off  latency=0  reg_retiming=on  dbl_ovrd=off  block_type=delay
  reint1 : xbsIndex_r4/Reinterpret  force_arith_type=on  arith_type=Unsigned  force_bin_pt=on  bin_pt=0  block_type=reinterpret
  sim_out : Terminator
  sim_out_reg_gw : xbsIndex_r4/Gateway Out  inherit_from_input=off  hdl_port=off  rows=1  columns=1  UseAsDAC=off  DACChannel='1'  interface=None  automatic_assignment=on  address_offset=hex2dec('00')  intf_name=''  intf_description=''  timing_constraint=None  locs_specified=off  LOCs={}  io_standard={}  block_type=gatewayout
  sim_out_reg_sim_delay : xbsIndex_r4/Delay  rst=off  infoeditControl=Selection of Reset will increase slice count due to use of real FFs and instead of SRLs  en=off  latency=1  reg_retiming=on  dbl_ovrd=off  block_type=delay
  souk_single_pipeline_4x2_common_autocorr_acc_cnt_user_data_in : xbsIndex_r4/Gateway Out  inherit_from_input=off  hdl_port=on  rows=1  columns=1  UseAsDAC=off  DACChannel='1'  interface=None  automatic_assignment=on  address_offset=hex2dec('00')  intf_name=''  intf_description=''  timing_constraint=None  locs_specified=off  LOCs={}  io_standard={}  block_type=gatewayout
  sim_out_reg : Outport  VectorParamsAs1DForOutWhenUnconnected=off
  wires:
  sim_out_reg_sim_delay/1 -> sim_out_reg_gw/1
  sim_out_reg_gw/1 -> sim_out_reg/1
  io_delay/1 -> cast_gw/1
  cast_gw/1 -> souk_single_pipeline_4x2_common_autocorr_acc_cnt_user_data_in/1
  souk_single_pipeline_4x2_common_autocorr_acc_cnt_user_data_in/1 -> sim_out/1
  out_reg/1 -> sim_out_reg_sim_delay/1, assert_reg/1
  assert_reg/1 -> reint1/1
  reint1/1 -> io_delay/1

== system souk_single_pipeline_4x2/common/autocorr/acc_len ==
  sim_1 : Inport
  convert1_1 : DataTypeConversion  OutDataTypeStr=fixdt('ufix32_En0')  LockScale=on
  convert2_1 : DataTypeConversion  OutDataTypeStr=fixdt('ufix32_En0')  ConvertRealWorld=Stored Integer (SI)  LockScale=on
  gain_1 : Gain  OutDataTypeStr=fixdt('ufix32_En0')
  io_delay : xbsIndex_r4/Delay  rst=off  infoeditControl=Selection of Reset will increase slice count due to use of real FFs and instead of SRLs  en=off  latency=0  reg_retiming=on  dbl_ovrd=off  block_type=delay
  reint1 : xbsIndex_r4/Reinterpret  force_arith_type=on  arith_type=Unsigned  force_bin_pt=on  bin_pt=0  block_type=reinterpret
  slice_reg : xbsIndex_r4/Slice  nbits=32  boolean_output=off  mode=Lower Bit Location + Width  bit1=0  base1=MSB of Input  bit0=0  base0=LSB of Input  dbl_ovrd=off  block_type=slice
  souk_single_pipeline_4x2_common_autocorr_acc_len_user_data_out : xbsIndex_r4/Gateway In  gui_display_data_type=Fixed-point  arith_type=Unsigned  n_bits=32  bin_pt=0  preci_type=Single  exp_width=8  frac_width=24  rows=1  columns=1  quantization="Round  (unbiased: +/- Inf)"  overflow=Saturate  period=1  UseAsADC=off  ADCChannel='1'  interface=None  automatic_assignment=on  address_offset=hex2dec('00')  intf_name=''  intf_description=''  default_value=0  timing_constraint=None  locs_specified=off  LOCs={}  io_standard={}  inherit_from_input=off  hdl_port=on  dbl_ovrd=off  block_type=gatewayin
  in_reg : Outport  VectorParamsAs1DForOutWhenUnconnected=off
  wires:
  souk_single_pipeline_4x2_common_autocorr_acc_len_user_data_out/1 -> io_delay/1
  sim_1/1 -> convert1_1/1
  convert1_1/1 -> convert2_1/1
  convert2_1/1 -> gain_1/1
  gain_1/1 -> souk_single_pipeline_4x2_common_autocorr_acc_len_user_data_out/1
  io_delay/1 -> slice_reg/1
  slice_reg/1 -> reint1/1
  reint1/1 -> in_reg/1

== system souk_single_pipeline_4x2/common/autocorr/trig ==
  sim_1 : Inport
  convert1_1 : DataTypeConversion  OutDataTypeStr=fixdt('ufix1_En0')  LockScale=on
  convert2_1 : DataTypeConversion  OutDataTypeStr=fixdt('ufix1_En0')  ConvertRealWorld=Stored Integer (SI)  LockScale=on
  gain_1 : Gain  OutDataTypeStr=fixdt('ufix32_En0')
  io_delay : xbsIndex_r4/Delay  rst=off  infoeditControl=Selection of Reset will increase slice count due to use of real FFs and instead of SRLs  en=off  latency=0  reg_retiming=on  dbl_ovrd=off  block_type=delay
  slice_reg : xbsIndex_r4/Slice  nbits=1  boolean_output=on  mode=Lower Bit Location + Width  bit1=0  base1=MSB of Input  bit0=0  base0=LSB of Input  dbl_ovrd=off  block_type=slice
  souk_single_pipeline_4x2_common_autocorr_trig_user_data_out : xbsIndex_r4/Gateway In  gui_display_data_type=Fixed-point  arith_type=Unsigned  n_bits=32  bin_pt=0  preci_type=Single  exp_width=8  frac_width=24  rows=1  columns=1  quantization="Round  (unbiased: +/- Inf)"  overflow=Saturate  period=1  UseAsADC=off  ADCChannel='1'  interface=None  automatic_assignment=on  address_offset=hex2dec('00')  intf_name=''  intf_description=''  default_value=0  timing_constraint=None  locs_specified=off  LOCs={}  io_standard={}  inherit_from_input=off  hdl_port=on  dbl_ovrd=off  block_type=gatewayin
  in_reg : Outport  VectorParamsAs1DForOutWhenUnconnected=off
  wires:
  souk_single_pipeline_4x2_common_autocorr_trig_user_data_out/1 -> io_delay/1
  sim_1/1 -> convert1_1/1
  convert1_1/1 -> convert2_1/1
  convert2_1/1 -> gain_1/1
  gain_1/1 -> souk_single_pipeline_4x2_common_autocorr_trig_user_data_out/1
  io_delay/1 -> slice_reg/1
  slice_reg/1 -> in_reg/1
